simulink model "btson"  (R2016a)
settings: Solver=ode5  StartTime=0.0  StopTime=4000.0  FixedStep=0.01  RelTol=1e-3
undefined symbols (not defined in the file): sigbuilder_block
libraries: fuzblock x1
settings Model: Creator=DELL  LastModifiedBy=DELL

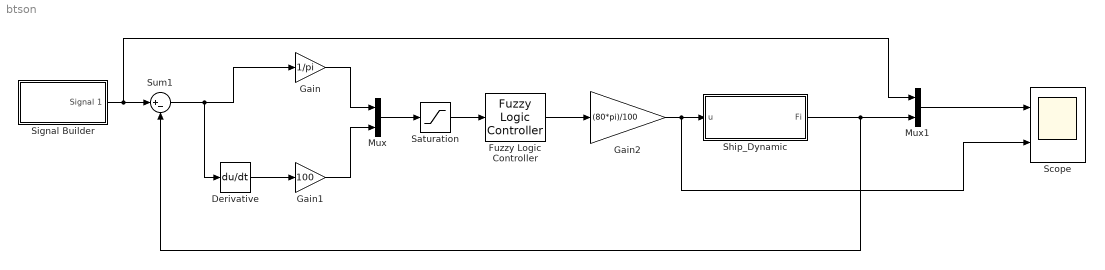
== system btson ==
  Derivative : Derivative
  Fuzzy Logic Controller : fuzblock/Fuzzy Logic  Controller  fis='bt1.fis'
  Gain : Gain  Gain=1/pi
  Gain1 : Gain  Gain=100
  Gain2 : Gain  Gain=(80*pi)/100
  Mux : Mux  Inputs=2
  Mux1 : Mux  Inputs=2
  Saturation : Saturate  UpperLimit=1  LowerLimit=-1
  Scope : Scope  NumInputPorts=2
  Ship_Dynamic : Subsystem  TreatAsAtomicUnit=on  mask{k=-0.12, t_1=0.176, t_2=0.0118, t_3=0.028}
  Signal Builder : Subsystem  Tag=STV Subsys  LoadFcn=sigbuilder_block('load');  StartFcn=sigbuilder_block('start');  StopFcn=sigbuilder_block('stop');  ClipboardFcn=sigbuilder_block('clipboard');  mask(Sigbuilder block){}
      mask help: Simulink:masks:SigbuilderBlock_MD
      mask init:
      | if ~strcmp(get_param(bdroot(gcbh),'SimulationStatus'),'stopped') tuvar = sigbuilder_block('maskInit'); end
      settings: CopyFcn=sigbuilder_block('copy');  DeleteFcn=sigbuilder_block('delete');  ModelCloseFcn=sigbuilder_block('modelClose');  PreSaveFcn=sigbuilder_block('preSave');  PauseFcn=sigbuilder_block('pause');  ContinueFcn=sigbuilder_block('continue');  NameChangeFcn=sigbuilder_block('namechange');  OpenFcn=sigbuilder_block('open',[437.6 199.2 550.4 400 ]);  CloseFcn=sigbuilder_block('close');
      mask Display: plot(0, 0, 100, 100,[2, 2, 32, 32, 2], [68, 8, 8, 68, 68],[32, 2], [38, 38], [32, 19, 2],[53, 60, 44], [32, 17, 17, 2],[16, 16, 31, 31]);txt = getActiveGroup(gcbh);text(2, 100, txt,'verticalAlignment', 'top');
  Sum1 : Sum  Inputs=|+-
  wires:
  Mux1/1 -> Scope/1
  Ship_Dynamic/1(Fi) -> Mux1/2, Sum1/2
  Gain2/1 -> Ship_Dynamic/1(u), Scope/2
  Mux/1 -> Saturation/1
  Saturation/1 -> Fuzzy Logic Controller/1
  Gain1/1 -> Mux/2
  Gain/1 -> Mux/1
  Fuzzy Logic Controller/1 -> Gain2/1
  Sum1/1 -> Derivative/1, Gain/1
  Derivative/1 -> Gain1/1
  Signal Builder/1(Signal 1) -> Mux1/1, Sum1/1

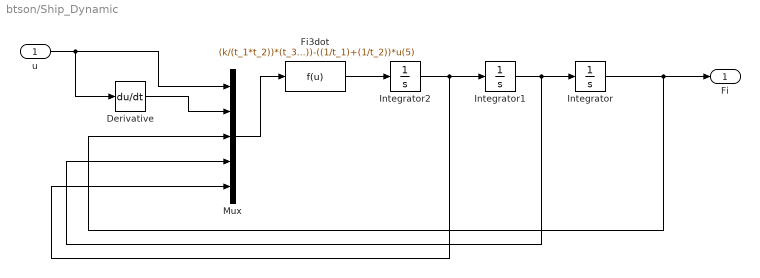
== system btson/Ship_Dynamic ==
  u : Inport
  Derivative : Derivative
  Fi3dot : Fcn  Expr=(k/(t_1*t_2))*(t_3*u(2)+u(1))-(1/(t_1*t_2))*(((u(4))^3)+u(4))-((1/t_1)+(1/t_2))*u(5)
  Integrator : Integrator
  Integrator1 : Integrator
  Integrator2 : Integrator
  Mux : Mux  Inputs=5
  Fi : Outport
  wires:
  Integrator/1 -> Mux/3, Fi/1
  Integrator1/1 -> Mux/4, Integrator/1
  Integrator2/1 -> Mux/5, Integrator1/1
  u/1 -> Derivative/1, Mux/1
  Derivative/1 -> Mux/2
  Fi3dot/1 -> Integrator2/1
  Mux/1 -> Fi3dot/1

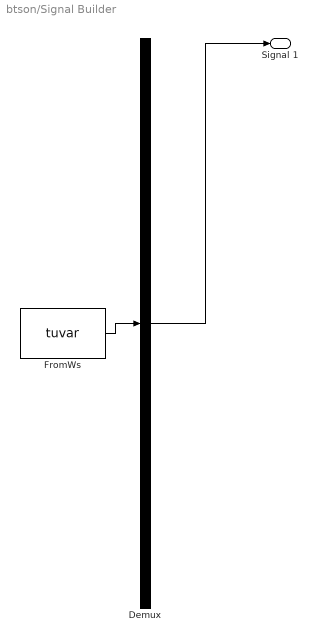
== system btson/Signal Builder ==
  Demux : Demux  Tag=STV Demux  Outputs=1
  FromWs : FromWorkspace  Tag=STV FromWs  VariableName=tuvar  SampleTime=0
      SigBuilderData=|
      | common.afterFinalStr = 'Extrapolate'
      | common.sampleTime = 0
      | dataSet.timeRange = [0 4000]
      | dataSet.name = 'Group 1'
      | sbobj.Groups.Name = 'Group 1'
      | sbobj.Groups.Signals.Name = 'Signal 1'
      | sbobj.Groups.Signals.XData = [0 4 6 500 500 1540 1540 3060 3060 4000]
      | sbobj.Groups.Signals.YData = [0 0 0 0 0.9 0.9 0.68 0.68 0.37 0.37]
      | sbobj.Groups.TimeRange = [0 4000]
  Signal 1 : Outport  Tag=STV Outport
  wires:
  Demux/1 -> Signal 1/1
  FromWs/1 -> Demux/1
